simulink model "Model_plant_Hpass"  (R2022a)
settings: Solver=ode45  StartTime=0.0  StopTime=20  RelTol=1e-3
values from neighbouring files (symbols this model uses):
  A = [0 0 1 0 0 ... (first row only)    [DesignProjectP2.m]    (also in DesignProjectP3.m; DesignProject_OffsetP3.m; mpc_example_regulation.m = [ 	 0,       0,              1,  0, 0; 	 0,       0,        ; mpc_example_tracking.m = [ 	 0,       0,              1,  0, 0; 	 0,       0,        )
  B = [0;0;0;0;1/La]    [DesignProjectP2.m]    (also in DesignProjectP3.m; DesignProject_OffsetP3.m; mpc_example_regulation.m = [0; 0; 0; 0; 1/La]; mpc_example_tracking.m = [0; 0; 0; 0; 1/La])
  C = [0 1 0 0 0]    [DesignProjectP2.m]    (also in DesignProjectP3.m = [1 0 0 0 0; DesignProject_OffsetP3.m = [1 0 0 0 0; mpc_example_regulation.m = [1 0 0 0 0; mpc_example_tracking.m = [1 0 0 0 0)
  D = 0    [DesignProjectP2.m]    (also in DesignProjectP3.m; DesignProject_OffsetP3.m; phase2_emc.m = zeros(sizeC(1),sizeB(2)))
  init = [theta_m_init; theta_l_init; thetadot_m_init; thetadot_l_init; Ia_init]    [ELEN90064_Project_Parameters.m]
  theta_l_init = deg2rad(30)    [ELEN90064_Project_Parameters.m]    (also in mpc_example_regulation.m = deg2rad(0); mpc_example_tracking.m = deg2rad(0))
  vision_fps = 50    [ELEN90064_Project_Parameters.m]
undefined symbols (not defined in the file or in its folder): denC, denEuler, denLPEuler, denLPTustin, denLPZOH, denTustin, denZOH, numC, numEuler, numLPEuler, numLPTustin, numLPZOH, numTustin, numZOH, w0
settings Model: Creator=Admin  LastModifiedBy=Admin

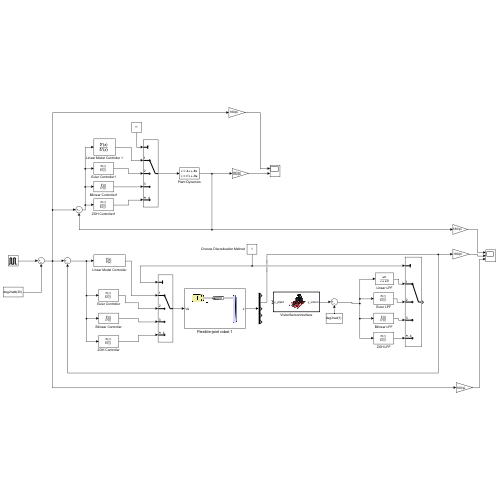
[thumbnail: Simulink's stored preview of the top-level diagram]
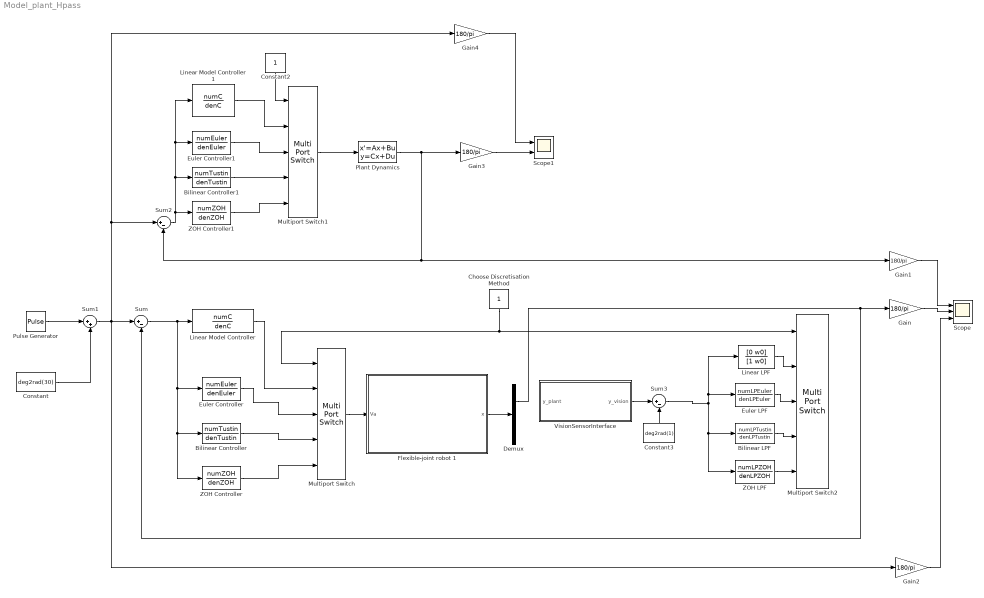
== system Model_plant_Hpass ==
  Bilinear Controller : DiscreteTransferFcn  Numerator=numTustin  Denominator=denTustin
  Bilinear Controller1 : DiscreteTransferFcn  Numerator=numTustin  Denominator=denTustin
  Bilinear LPF : DiscreteTransferFcn  Numerator=numLPTustin  Denominator=denLPTustin
  Choose Discretisation Method : Constant
  Constant : Constant  Value=deg2rad(30)
  Constant2 : Constant
  Constant3 : Constant  Value=deg2rad(1)
  Demux : Demux  Outputs=5
  Euler Controller : DiscreteTransferFcn  Numerator=numEuler  Denominator=denEuler
  Euler Controller1 : DiscreteTransferFcn  Numerator=numEuler  Denominator=denEuler
  Euler LPF : DiscreteTransferFcn  Numerator=numLPEuler  Denominator=denLPEuler
  Flexible-joint robot 1 : Subsystem
      mask Display: image('$imagefile'); % Use "Edit Image" on toolstrip to change.
  Gain{,1..4} (5 alike) : Gain  Gain=180/pi
  Linear LPF : TransferFcn  Numerator=[0 w0]  Denominator=[1 w0]
  Linear Model Controller : TransferFcn  Numerator=numC  Denominator=denC
  Linear Model Controller 1 : TransferFcn  Numerator=numC  Denominator=denC
  Multiport Switch : MultiPortSwitch  Inputs=4  SaturateOnIntegerOverflow=off  InputSameDT=off
  Multiport Switch1 : MultiPortSwitch  Inputs=4  SaturateOnIntegerOverflow=off  InputSameDT=off
  Multiport Switch2 : MultiPortSwitch  Inputs=4  SaturateOnIntegerOverflow=off  InputSameDT=off
  Plant Dynamics : StateSpace  A=A  B=B  C=C  D=D  InitialCondition=deg2rad(30)
  Pulse Generator : DiscretePulseGenerator  PulseType=Time based  Amplitude=deg2rad(30)  Period=10  PulseWidth=50
  Scope : Scope  NumInputPorts=3
  Scope1 : Scope  NumInputPorts=2
  Sum : Sum  Inputs=|+-
  Sum1 : Sum  Inputs=|++
  Sum2 : Sum  Inputs=|+-
  Sum3 : Sum  Inputs=|+-
  VisionSensorInterface : Subsystem  TreatAsAtomicUnit=on
      mask Display: image('$imagefile'); % Use "Edit Image" on toolstrip to change.
  ZOH Controller : DiscreteTransferFcn  Numerator=numZOH  Denominator=denZOH
  ZOH Controller1 : DiscreteTransferFcn  Numerator=numZOH  Denominator=denZOH
  ZOH LPF : DiscreteTransferFcn  Numerator=numLPZOH  Denominator=denLPZOH
  wires:
  Sum/1 -> ZOH Controller/1, Bilinear Controller/1, Euler Controller/1, Linear Model Controller/1
  Pulse Generator/1 -> Sum1/1
  Constant/1 -> Sum1/2
  Gain/1 -> Scope/2
  Flexible-joint robot 1/1(x) -> Demux/1
  Plant Dynamics/1 -> Gain1/1, Sum2/2, Gain3/1
  Sum1/1 -> Sum/1, Gain2/1, Sum2/1, Gain4/1
  Gain1/1 -> Scope/1
  Gain2/1 -> Scope/3
  Sum3/1 -> Linear LPF/1, Euler LPF/1, ZOH LPF/1, Bilinear LPF/1
  Demux/2 -> Gain/1, Sum/2
  Linear Model Controller/1 -> Multiport Switch/2
  Euler Controller/1 -> Multiport Switch/3
  Bilinear Controller/1 -> Multiport Switch/4
  ZOH Controller/1 -> Multiport Switch/5
  Choose Discretisation Method/1 -> Multiport Switch/1, Multiport Switch2/1
  Multiport Switch/1 -> Flexible-joint robot 1/1(Va)
  Sum2/1 -> ZOH Controller1/1, Linear Model Controller 1/1, Euler Controller1/1, Bilinear Controller1/1
  Linear Model Controller 1/1 -> Multiport Switch1/2
  Euler Controller1/1 -> Multiport Switch1/3
  Bilinear Controller1/1 -> Multiport Switch1/4
  ZOH Controller1/1 -> Multiport Switch1/5
  Constant2/1 -> Multiport Switch1/1
  Multiport Switch1/1 -> Plant Dynamics/1
  Gain3/1 -> Scope1/2
  Gain4/1 -> Scope1/1
  Linear LPF/1 -> Multiport Switch2/2
  Euler LPF/1 -> Multiport Switch2/3
  Bilinear LPF/1 -> Multiport Switch2/4
  ZOH LPF/1 -> Multiport Switch2/5
  Constant3/1 -> Sum3/2
  VisionSensorInterface/1(y_vision) -> Sum3/1

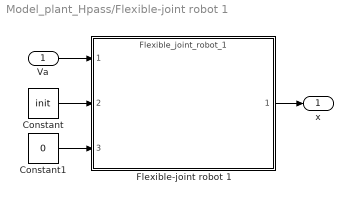
== system Model_plant_Hpass/Flexible-joint robot 1 ==
  Va : Inport
  Constant : Constant  Value=init
  Constant1 : Constant  Value=0
  Flexible-joint robot 1 : ModelReference  ModelNameDialog=Flexible_joint_robot_1  ModelReferenceVersion=1.65  CopyOfModelProtected=on
  x : Outport
  wires:
  Constant/1 -> Flexible-joint robot 1/2
  Constant1/1 -> Flexible-joint robot 1/3
  Flexible-joint robot 1/1 -> x/1
  Va/1 -> Flexible-joint robot 1/1

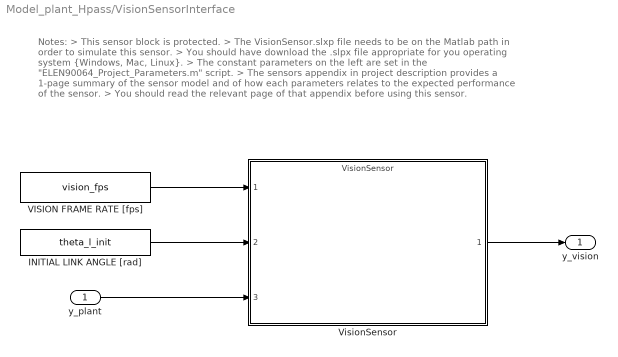
== system Model_plant_Hpass/VisionSensorInterface ==
  note: Notes:
      | > This sensor block is protected.
      | > The VisionSensor.slxp file needs to be on the Matlab path in order to simulate this sensor.
      | > You should have download the .slpx file appropriate for you operating system {Windows, Mac, Linux}.
      | > The constant parameters on the left are set in the "ELEN90064_Project_Parameters.m" script.
      | > The sensors appendix in project description provides a 1-page summary of the sensor model and of how each parameters relates to the expected performance of the sensor.
      | > You should read the relevant page of that appendix before using this sensor.
  y_plant : Inport
  INITIAL LINK ANGLE [rad] : Constant  Value=theta_l_init
  VISION FRAME RATE [fps] : Constant  Value=vision_fps
  VisionSensor : ModelReference  ModelNameDialog=VisionSensor.slxp  ModelReferenceVersion=1.19  CopyOfModelProtected=on
  y_vision : Outport
  wires:
  VISION FRAME RATE [fps]/1 -> VisionSensor/1
  INITIAL LINK ANGLE [rad]/1 -> VisionSensor/2
  y_plant/1 -> VisionSensor/3
  VisionSensor/1 -> y_vision/1
